simulink model "stavova_zv_model"  (R2014b)
settings: Solver=ode45  StartTime=0.0  StopTime=10.0  RelTol=1e-3
values from neighbouring files (symbols this model uses):
  Alin = eval(Alin)    [main.m]    (also in matlab.mat = [0 0 0 0 0 0 14.3782406735 -97.1270102365 1 0 -8.0820897902 ; stav_lin.mat = [0 0 0 0 0 0 5.28235362921 -73.758221558 1 0 -6.9230827764 9; stavova_zpetna.m; workspace.mat = [0 0 0 0 0 0 5.28235362921 -73.758221558 1 0 -6.9230827764 9)
  b = ku/k    [glabatom.m]    (also in matlab.mat = 0.251206720988)
  Blin = eval(Blin)    [main.m]    (also in matlab.mat = [0 0 32.1730635168 -49.2662800726]; stav_lin.mat = [0 0 13.3327451106 -18.0997049117]; stavova_zpetna.m; workspace.mat = [0 0 13.3327451106 -18.0997049117])
  Clin = eval(Clin)    [main.m]    (also in matlab.mat = [1  0  0  0; 0  1  0  0]; stavova_zpetna.m; workspace.mat = [1  0  0  0; 0  1  0  0])
  delta = Jp*zeta*omegan    [glabatom.m]    (also in matlab.mat = 0.000181694248674)
  Dlin = eval(Dlin)    [main.m]    (also in matlab.mat = [0 0]; stavova_zpetna.m; workspace.mat = [0 0])
  Jp = m*g*l/(omegan^2)    [glabatom.m]    (also in matlab.mat = 0.00388561360108)
  K = acker(Alin, Blin,P)    [stavova_zpetna.m]
  k1 = T*b    [main.m]    (also in matlab.mat = 0.0401930753581; stavova_zpetna.m)
  k2 = eval(k2)    [main.m]    (also in matlab.mat = 0.00595; stavova_zpetna.m)
  k3 = eval(k3)    [main.m]    (also in matlab.mat = 0.2918475; stavova_zpetna.m)
  ku = 16    [main.m]    (also in matlab.mat = 8; stavova_zpetna.m)
  up1 = 0    [main.m]    (also in matlab.mat; stavova_zpetna.m)
  x1p = 0    [main.m]    (also in matlab.mat; stavova_zpetna.m)
  x2p = -pi/2    (= -1.57079632679)    [main.m]    (also in matlab.mat; stavova_zpetna.m = 1.57079632679)
  x3p = 0    [main.m]    (also in matlab.mat; stavova_zpetna.m)
  x4p = 0    [main.m]    (also in matlab.mat; stavova_zpetna.m)
  y1p = 0    [main.m]    (also in matlab.mat; stavova_zpetna.m)
  y2p = -pi/2    (= -1.57079632679)    [main.m]    (also in matlab.mat; stavova_zpetna.m)
settings Model: Creator=glab  LastModifiedBy=glab

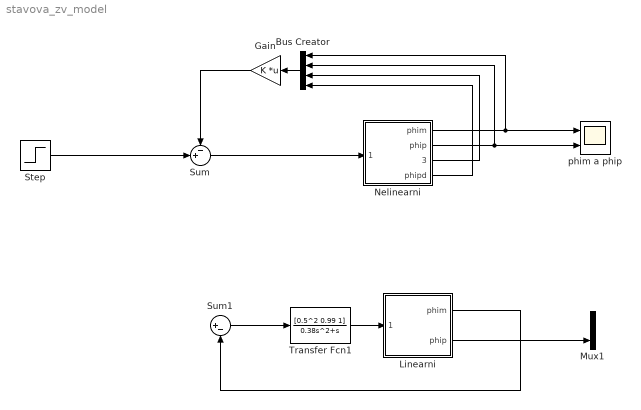
== system stavova_zv_model ==
  Bus Creator : BusCreator
  Gain : Gain  Gain=K  Multiplication=Matrix(K*u)
  Linearni : Subsystem
  Mux1 : Mux  Inputs=2
  Nelinearni : Subsystem
  Step : Step  Time=0  After=pi/2  SampleTime=0
  Sum : Sum  Inputs=-+|
  Sum1 : Sum  Inputs=|+-
  Transfer Fcn1 : TransferFcn  Numerator=[0.5^2 0.99 1]  Denominator=[0.38 1 0]
  phim a phip : Scope  NumInputPorts=2
      settings: ShowLegends=on  YMin=-5~-5  YMax=5~5  SaveName=vystup
  wires:
  Linearni/1(phim) -> Sum1/2
  Nelinearni/1(phim) -> phim a phip/1, Bus Creator/1
  Linearni/2(phip) -> Mux1/2
  Nelinearni/2(phip) -> phim a phip/2, Bus Creator/2
  Sum/1 -> Nelinearni/1(u_norm)
  Sum1/1 -> Transfer Fcn1/1
  Transfer Fcn1/1 -> Linearni/1(u_norm)
  Step/1 -> Sum/2
  Nelinearni/3(phimd) -> Bus Creator/3
  Nelinearni/4(phipd) -> Bus Creator/4
  Bus Creator/1 -> Gain/1
  Gain/1 -> Sum/1

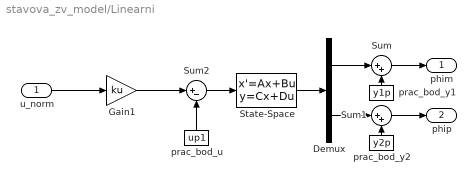
== system stavova_zv_model/Linearni ==
  u_norm : Inport
  Demux : Demux  Outputs=2
  Gain1 : Gain  Gain=ku
  State-Space : StateSpace  A=Alin  B=Blin  C=Clin  D=Dlin  X0=0
  Sum : Sum  Inputs=|++
  Sum1 : Sum  Inputs=|++
  Sum2 : Sum  Inputs=|+-
  prac_bod_u : Constant  Value=up1
  prac_bod_y1 : Constant  Value=y1p
  prac_bod_y2 : Constant  Value=y2p
  phim : Outport
  phip : Outport  Port=2
  wires:
  State-Space/1 -> Demux/1
  Demux/1 -> Sum/1
  prac_bod_y1/1 -> Sum/2
  Sum/1 -> phim/1
  prac_bod_y2/1 -> Sum1/2
  Sum1/1 -> phip/1
  Demux/2 -> Sum1/1
  u_norm/1 -> Gain1/1
  prac_bod_u/1 -> Sum2/2
  Sum2/1 -> State-Space/1
  Gain1/1 -> Sum2/1

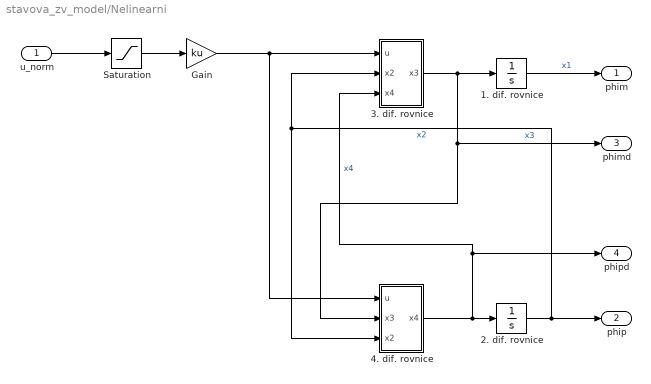
== system stavova_zv_model/Nelinearni ==
  u_norm : Inport
  1. dif. rovnice : Integrator  InitialCondition=x1p
  2. dif. rovnice : Integrator  InitialCondition=x2p
  3. dif. rovnice : Subsystem
  4. dif. rovnice : Subsystem
  Gain : Gain  Gain=ku
  Saturation : Saturate  UpperLimit=1  LowerLimit=-1
  phim : Outport
  phip : Outport  Port=2
  phimd : Outport  Port=3
  phipd : Outport  Port=4
  wires:
  1. dif. rovnice/1 -> phim/1  "x1"
  4. dif. rovnice/1(x4) -> phipd/1, 3. dif. rovnice/3(x4), 2. dif. rovnice/1  "x4"
  2. dif. rovnice/1 -> phip/1, 4. dif. rovnice/3(x2), 3. dif. rovnice/2(x2)  "x2"
  3. dif. rovnice/1(x3) -> 4. dif. rovnice/2("x3 "), phimd/1, 1. dif. rovnice/1  "x3"
  u_norm/1 -> Saturation/1
  Gain/1 -> 4. dif. rovnice/1(u), 3. dif. rovnice/1(u)
  Saturation/1 -> Gain/1

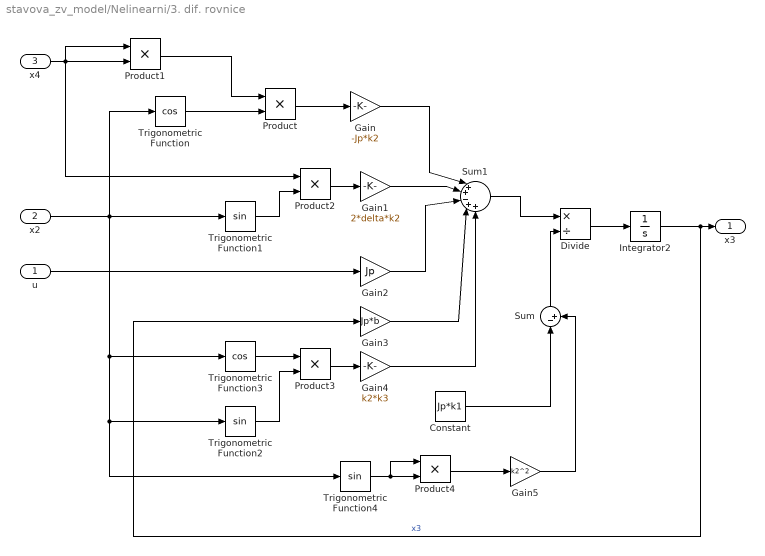
== system stavova_zv_model/Nelinearni/3. dif. rovnice ==
  u : Inport
  x2 : Inport  Port=2
  x4 : Inport  Port=3
  Constant : Constant  Value=Jp*k1
  Divide : Product  Inputs=*/
  Gain : Gain  Gain=-Jp*k2
  Gain1 : Gain  Gain=2*delta*k2
  Gain2 : Gain  Gain=Jp
  Gain3 : Gain  Gain=Jp*b
  Gain4 : Gain  Gain=k2*k3
  Gain5 : Gain  Gain=k2^2
  Integrator2 : Integrator  InitialCondition=x3p
  Product{,1..4} (5 alike) : Product
  Sum : Sum  Inputs=|-+
  Sum1 : Sum  Inputs=|++-++
  Trigonometric Function : Trigonometry  Operator=cos
  Trigonometric Function1 : Trigonometry
  Trigonometric Function2 : Trigonometry
  Trigonometric Function3 : Trigonometry  Operator=cos
  Trigonometric Function4 : Trigonometry
  x3 : Outport
  wires:
  Trigonometric Function3/1 -> Product3/1
  Divide/1 -> Integrator2/1
  x2/1 -> Trigonometric Function4/1, Trigonometric Function2/1, Trigonometric Function3/1, Trigonometric Function1/1, Trigonometric Function/1
  Product3/1 -> Gain4/1
  Trigonometric Function2/1 -> Product3/2
  Gain4/1 -> Sum1/5
  Gain/1 -> Sum1/1
  Product2/1 -> Gain1/1
  Trigonometric Function1/1 -> Product2/2
  u/1 -> Gain2/1
  Gain3/1 -> Sum1/4
  Gain1/1 -> Sum1/2
  Gain2/1 -> Sum1/3
  Sum1/1 -> Divide/1
  Product/1 -> Gain/1
  Sum/1 -> Divide/2
  x4/1 -> Product1/2, Product2/1, Product1/1
  Product1/1 -> Product/1
  Integrator2/1 -> Gain3/1, x3/1  "x3"
  Trigonometric Function/1 -> Product/2
  Gain5/1 -> Sum/2
  Constant/1 -> Sum/1
  Product4/1 -> Gain5/1
  Trigonometric Function4/1 -> Product4/1, Product4/2

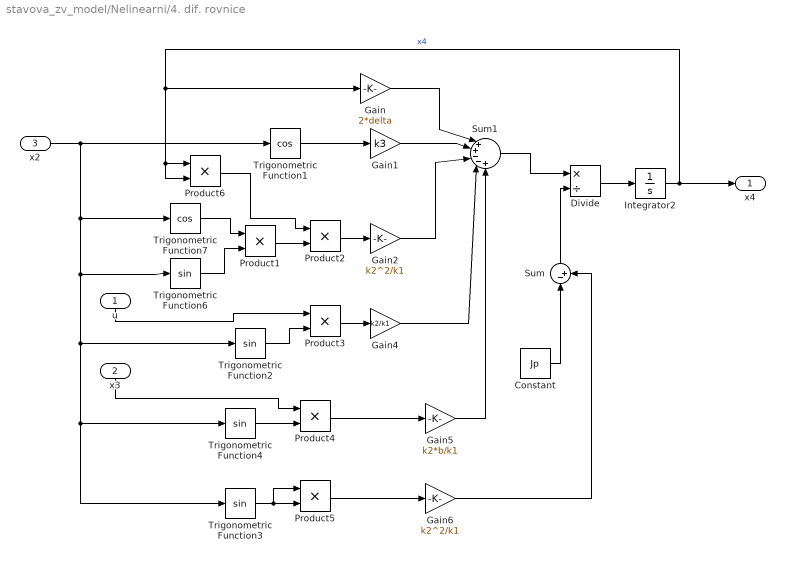
== system stavova_zv_model/Nelinearni/4. dif. rovnice ==
  u : Inport
  "x3 " : Inport  Port=2
  x2 : Inport  Port=3
  Constant : Constant  Value=Jp
  Divide : Product  Inputs=*/
  Gain : Gain  Gain=2*delta
  Gain1 : Gain  Gain=k3
  Gain2 : Gain  Gain=k2^2/k1
  Gain4 : Gain  Gain=k2/k1
  Gain5 : Gain  Gain=k2*b/k1
  Gain6 : Gain  Gain=k2^2/k1
  Integrator2 : Integrator  InitialCondition=x4p
  Product{1..6} (6 alike) : Product
  Sum : Sum  Inputs=|-+
  Sum1 : Sum  Inputs=|++--+
  Trigonometric Function1 : Trigonometry  Operator=cos
  Trigonometric Function{2..4,6} (4 alike) : Trigonometry
  Trigonometric Function7 : Trigonometry  Operator=cos
  x4 : Outport
  wires:
  Trigonometric Function3/1 -> Product5/1, Product5/2
  Product5/1 -> Gain6/1
  Divide/1 -> Integrator2/1
  Product3/1 -> Gain4/1
  Gain/1 -> Sum1/1
  Constant/1 -> Sum/1
  Gain6/1 -> Sum/2
  Integrator2/1 -> x4/1, Gain/1, Product6/1, Product6/2  "x4"
  Sum/1 -> Divide/2
  Product4/1 -> Gain5/1
  Sum1/1 -> Divide/1
  Gain2/1 -> Sum1/3
  Gain1/1 -> Sum1/2
  Trigonometric Function1/1 -> Gain1/1
  Trigonometric Function2/1 -> Product3/2
  Trigonometric Function6/1 -> Product1/2
  Trigonometric Function7/1 -> Product1/1
  Gain5/1 -> Sum1/5
  Trigonometric Function4/1 -> Product4/2
  Gain4/1 -> Sum1/4
  Product2/1 -> Gain2/1
  u/1 -> Product3/1
  x2/1 -> Trigonometric Function3/1, Trigonometric Function4/1, Trigonometric Function2/1, Trigonometric Function6/1, Trigonometric Function7/1, Trigonometric Function1/1
  "x3 "/1 -> Product4/1
  Product1/1 -> Product2/2
  Product6/1 -> Product2/1
